simulink model "control_wiht_motor"  (R2024b)
settings: Solver=FixedStepAuto  StartTime=0.0  StopTime=180  FixedStep=0.01  RelTol=1e-3
libraries: arduinolib x3, simulink x2
settings Model: ExtModeTrigDuration=2  Creator=USER  LastModifiedBy=USER
settings SolverCC: AutoInsertRateTranBlk=on
settings OptimizationCC: EnhancedBackFolding=on  PassReuseOutputArgsAs=Individual arguments  ZeroExternalMemoryAtStartup=off  ZeroInternalMemoryAtStartup=off  MaxStackSize=64  OptimizeBlockOrder=speed  DifferentSizesBufferReuse=on  OptimizationCustomize=off  EfficientTunableParamExpr=on
settings DebuggingCC: ParameterTunabilityLossMsg=error
settings HardwareCC: ProdBitPerInt=16  ProdBitPerPointer=16  ProdBitPerSizeT=16  ProdBitPerPtrDiffT=16  ProdLargestAtomicFloat=None  ProdWordSize=8  ProdHWDeviceType=Atmel->AVR
settings SFSimCC: MATLABDynamicMemAlloc=off
settings RTWCC: Description=Embedded Coder  SystemTargetFile=ert.tlc  HardwareBoard=Arduino Mega 2560  TemplateMakefile=ert_default_tmf  CustomHeaderCode="\"C:\\Users\\USER\\AppData\\Local\\Arduino15\\packages\\arduino\\hardware\\avr\\1.8.6\\cores\\arduino\\Arduino.h\""  Toolchain=Arduino AVR
settings CodeAppCC: ForceParamTrailComments=on  IgnoreCustomStorageClasses=off  OperatorAnnotations=on  SimulinkDataObjDesc=on  SFDataObjDesc=on  InsertBlockDesc=on
settings ERTTargetCC: SupportContinuousTime=on  SupportVariableSizeSignals=on  ExtModeTransport=3  ExtModeStaticAlloc=on  ExtModeAutomaticAllocSize=off  ExtModeStaticAllocSize=2048  ExtModeMexFile=ext_xcp  ExtModeIntrfLevel=Level2 - Open  InlinedParameterPlacement=Hierarchical

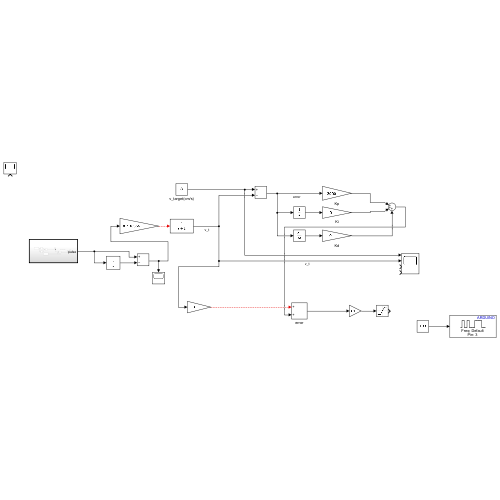
[thumbnail: Simulink's stored preview of the top-level diagram]
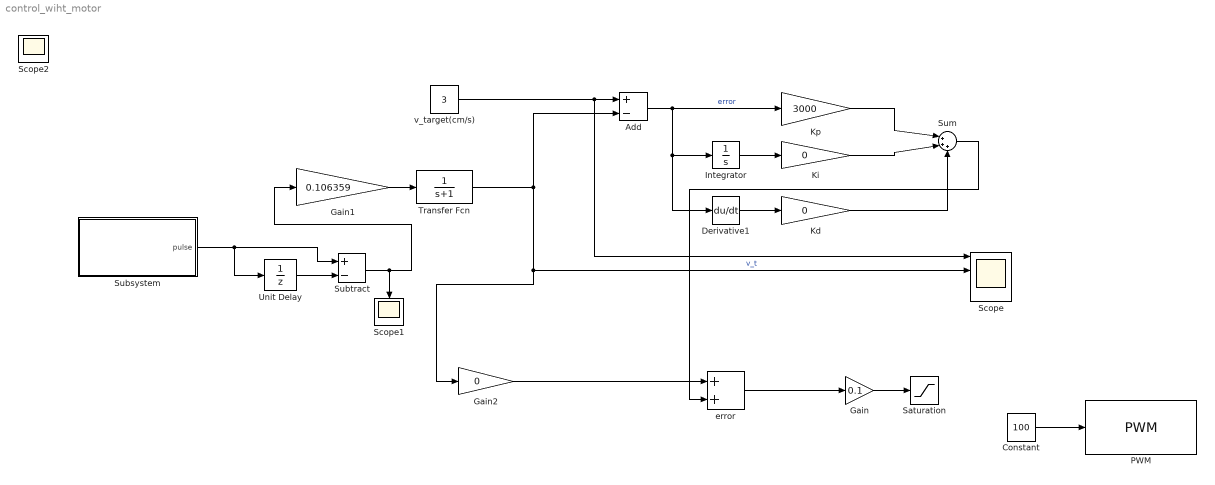
== system control_wiht_motor ==
  Add : Sum  Inputs=+-
  Constant : Constant  Value=100
  Derivative1 : Derivative
  Gain : Gain  Gain=0.1
  Gain1 : Gain  Gain=0.106359
  Gain2 : Gain  Gain=0
  Integrator : Integrator
  Kd : Gain  Gain=0
  Ki : Gain  Gain=0
  Kp : Gain  Gain=3000
  PWM : arduinolib/PWM  pinNumber=3  frequencyType=Default  desiredFrequency=490.2  achievableFrequency=490.2
      settings: SourceProductName=Common
  Saturation : Saturate  UpperLimit=255  LowerLimit=0
  Scope : Scope  NumInputPorts=4
  Scope1 : Scope
  Scope2 : Scope
  Subsystem : Subsystem  TreatAsAtomicUnit=on
  Subtract : Sum  Inputs=+-
  Sum : Sum  Inputs=|+++
  Transfer Fcn : TransferFcn  Denominator=[1 1]
  Unit Delay : UnitDelay  InitialCondition=10  SampleTime=-1  HasFrameUpgradeWarning=on
  error : Sum
  v_target(cm/s) : Constant  Value=3
  wires:
  v_target(cm/s)/1 -> Scope/1, Add/1
  Add/1 -> Derivative1/1, Integrator/1, Kp/1  "error"
  Gain2/1 -> error/1
  error/1 -> Gain/1
  Integrator/1 -> Ki/1
  Derivative1/1 -> Kd/1
  Kp/1 -> Sum/1
  Ki/1 -> Sum/2
  Kd/1 -> Sum/3
  Sum/1 -> error/2
  Gain/1 -> Saturation/1
  Gain1/1 -> Transfer Fcn/1
  Transfer Fcn/1 -> Add/2, Gain2/1, Scope/2  "v_t"
  Subtract/1 -> Scope1/1, Gain1/1
  Constant/1 -> PWM/1
  Subsystem/1(pulse) -> Unit Delay/1, Subtract/1
  Unit Delay/1 -> Subtract/2

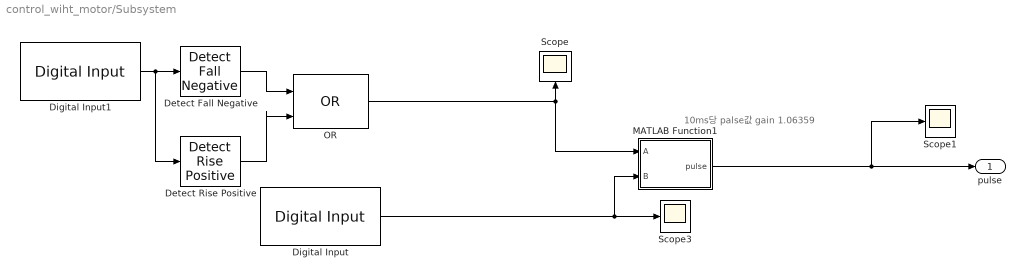
== system control_wiht_motor/Subsystem ==
  note: 10ms당 palse값 gain 1.06359
  Detect Fall Negative : simulink/Logic and Bit Operations/Detect Fall Negative  vinit=0  OutDataTypeStr=boolean
  Detect Rise Positive : simulink/Logic and Bit Operations/Detect Rise Positive  vinit=0  OutDataTypeStr=boolean
  Digital Input : arduinolib/Digital Input  pinNumber=2  mode=Default  Direction=input  SampleTime=0.1  blockPlatform=arduino
      settings: SourceProductName=Common
  Digital Input1 : arduinolib/Digital Input  pinNumber=4  mode=Default  Direction=input  SampleTime=0.1  blockPlatform=arduino
      settings: SourceProductName=Common
  MATLAB Function1 : MATLAB Function  TreatAsAtomicUnit=on
  OR : Logic  Operator=OR  IconShape=distinctive  AllPortsSameDT=off  OutDataTypeStr=boolean
  Scope : Scope
  Scope1 : Scope
  Scope3 : Scope
  pulse : Outport
  wires:
  OR/1 -> MATLAB Function1/1(A), Scope/1
  Digital Input1/1 -> Detect Rise Positive/1, Detect Fall Negative/1
  MATLAB Function1/1(pulse) -> pulse/1, Scope1/1
  Digital Input/1 -> MATLAB Function1/2(B), Scope3/1
  Detect Rise Positive/1 -> OR/2
  Detect Fall Negative/1 -> OR/1

== matlab function control_wiht_motor/Subsystem/MATLAB Function1 ==
  data: A input; B input; pulse output
function pulse = encoderLogic(A,B)
% A, B: logical (boolean) type
% pulse: int output

persistent prevA prevB pulseCount

if isempty(pulseCount)
    pulseCount = double(0);
    prevA = false;
    prevB = false;
end

if A ~= prevA
    pulseCount = pulseCount + 1;

end

prevA = A;
prevB = B;

pulse = pulseCount;
